simulink model "question8"  (R2018a)
settings: Solver=VariableStepAuto  StartTime=0.0  StopTime=10.0  RelTol=1e-3
PreLoadFcn:
  | load C:\Users\paul\Documents\lr\MSc\automatic flight control\assignment\code\github\FindF16Dynamics_q8.m
values from neighbouring files (symbols this model uses):
  A_new = A_lo([3 7 8 5 11],[3 7 8 5 11])    [FindF16Dynamics_q8.m]
  B_new = B_lo([3 7 8 5 11],1:2)    [FindF16Dynamics_q8.m]
  C_new = C_lo([3 7 8 5 11],[3 7 8 5 11])    [FindF16Dynamics_q8.m]
  D_new = D_lo([3 7 8 5 11],1:2)    [FindF16Dynamics_q8.m]
  elevator = minreal(transferfunctions(19,2))    [FindF16Dynamics.m]    (also in FindF16Dynamics_q5.m; FindF16Dynamics_q8.m = -0.09; runF16Sim.m = -0.09; runLINF16sim.m)
  LQR_matrix_outer = LQR_matrix(1,2:5)    [FindF16Dynamics_q8.m]
  thrust = 5000    [FindF16Dynamics.m]    (also in FindF16Dynamics_q5.m; FindF16Dynamics_q8.m; runF16Sim.m; runLINF16sim.m = 0)
undefined symbols (not defined in the file or in its folder): LQR_matrix_inner
settings Model: Creator=paul  LastModifiedBy=paul

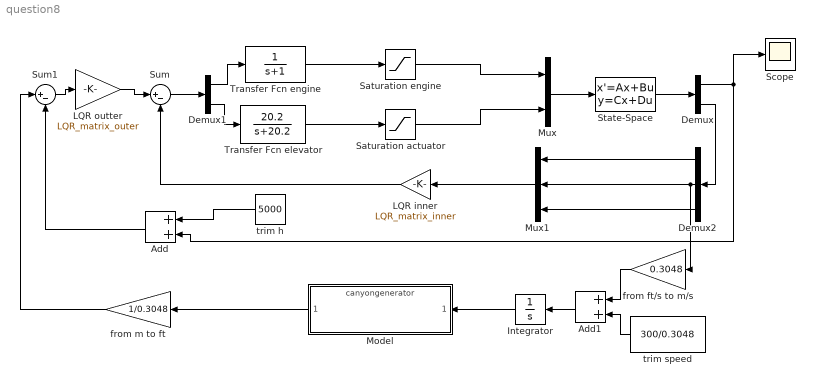
== system question8 ==
  Add : Sum
  Add1 : Sum
  Demux : Demux  Outputs=2
  Demux1 : Demux  Outputs=2
  Demux2 : Demux  Outputs=3
  Integrator : Integrator
  LQR inner : Gain  Gain=LQR_matrix_inner
  LQR outter : Gain  Gain=LQR_matrix_outer
  Model : ModelReference  ModelNameDialog=canyongenerator.mdl  SimulationMode=Normal  ModelReferenceVersion=1.7
  Mux : Mux  Inputs=2
  Mux1 : Mux  Inputs=3
  Saturation actuator : Saturate  UpperLimit=25-elevator  LowerLimit=-25-elevator
  Saturation engine : Saturate  UpperLimit=19000-thrust  LowerLimit=1000-thrust
  Scope : Scope
  State-Space : StateSpace  A=A_new  B=B_new  C=C_new  D=D_new  InitialCondition=[1/0.3048*1500;300;0;0;0]
  Sum : Sum  Inputs=|+-
  Sum1 : Sum  Inputs=|+-
  Transfer Fcn elevator : TransferFcn  Numerator=[20.2]  Denominator=[1 20.2]
  Transfer Fcn engine : TransferFcn  Denominator=[1 1]
  from ft/s to m/s : Gain  Gain=0.3048
  from m to ft : Gain  Gain=1/0.3048
  trim h : Constant  Value=5000
  trim speed : Constant  Value=300/0.3048
  wires:
  Transfer Fcn engine/1 -> Saturation engine/1
  Transfer Fcn elevator/1 -> Saturation actuator/1
  Saturation engine/1 -> Mux/1
  Saturation actuator/1 -> Mux/2
  Mux/1 -> State-Space/1
  State-Space/1 -> Demux/1
  Demux/1 -> Add/2, Scope/1
  Sum/1 -> Demux1/1
  Demux1/1 -> Transfer Fcn engine/1
  Demux1/2 -> Transfer Fcn elevator/1
  LQR inner/1 -> Sum/2
  LQR outter/1 -> Sum/1
  Sum1/1 -> LQR outter/1
  Demux/2 -> Demux2/1
  Demux2/1 -> Mux1/1
  Demux2/2 -> from ft/s to m/s/1, Mux1/2
  Demux2/3 -> Mux1/3
  Integrator/1 -> Model/1
  Mux1/1 -> LQR inner/1
  Add/1 -> Sum1/2
  Model/1 -> from m to ft/1
  from m to ft/1 -> Sum1/1
  trim h/1 -> Add/1
  Add1/1 -> Integrator/1
  from ft/s to m/s/1 -> Add1/1
  trim speed/1 -> Add1/2
